simulink model "hvdcmay22"  (R2024b)
settings: Solver=VariableStepAuto  StartTime=0.0  StopTime=0.5  RelTol=1e-3
undefined symbols (not defined in the file): D1, Delta, lagging, pulse
libraries: spsThreePhaseTransformerTwoWindingsLib x4, spsUniversalBridgeLib x4, spsThreePhaseVIMeasurementLib x3, spsMeanLib x2, spsPLL3phLib x2, spsPulseGeneratorThyristor12PulseLib x2, spsSeriesRLCBranchLib x2, spsThreePhaseSourceLib x2, spsCurrentMeasurementLib x1, spsThreePhaseHarmonicFilterLib x1, spsVoltageMeasurementLib x1, sps_lib x1
settings Model: Creator=HP  LastModifiedBy=HP
settings DataIOCC: SignalLogging=off  ReturnWorkspaceOutputs=off

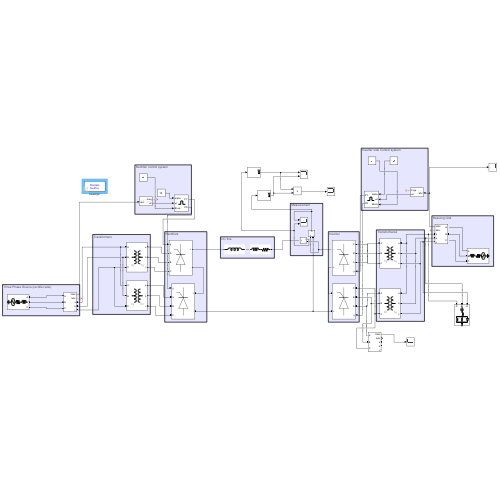
[thumbnail: Simulink's stored preview of the top-level diagram]
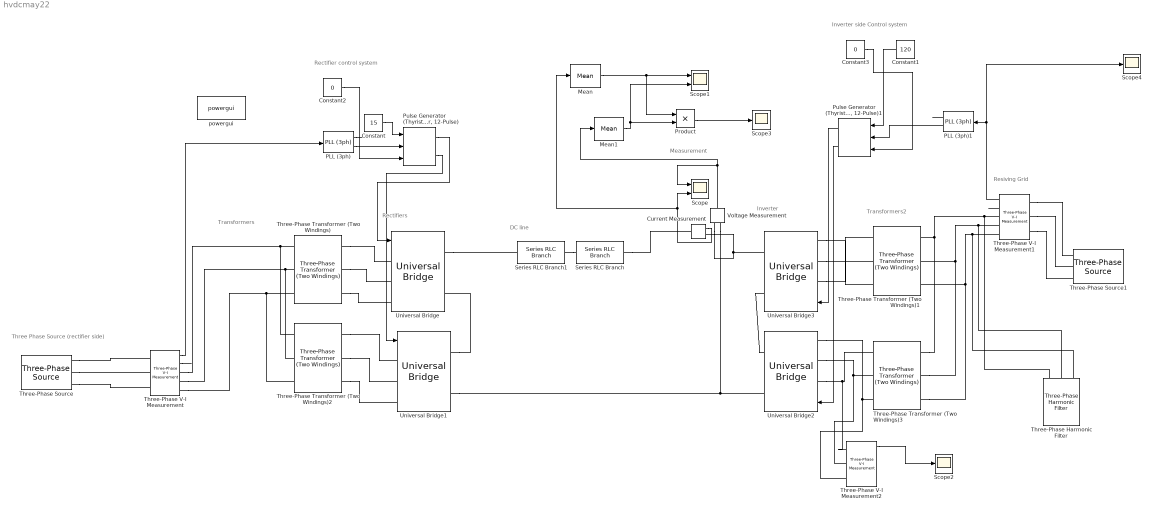
== system hvdcmay22 ==
  note: Transformers2
  note: Resiving Grid
  note: Inverter side Control system
  note: Measurement
  note: Inverter
  note: DC line
  note: Rectifiers
  note: Transformers
  note: Three Phase Source (rectifier side)
  note: Rectifier control system
  Constant : Constant  Value=15
  Constant1 : Constant  Value=120
  Constant2 : Constant  Value=0
  Constant3 : Constant  Value=0
  Current Measurement : spsCurrentMeasurementLib/Current Measurement  PhasorSimulation=off  OutputType=Complex  PSBequivalent=0
  Mean : spsMeanLib/Mean  Freq=60  Vinit=0  Ts=0
  Mean1 : spsMeanLib/Mean  Freq=60  Vinit=0  Ts=0
  PLL (3ph) : spsPLL3phLib/PLL (3ph)  Fmin=45  Par_Init=[0, 50]  ParK=[180, 3200, 1]  TcD=1e-4  MaxRateChangeFreq=12  FilterCutOffFreq=25  Ts=0  AGC=on
  PLL (3ph)1 : spsPLL3phLib/PLL (3ph)  Fmin=45  Par_Init=[0, 50]  ParK=[180, 3200, 1]  TcD=1e-4  MaxRateChangeFreq=12  FilterCutOffFreq=25  Ts=0  AGC=on
  Product : Product
  "Pulse Generator (Thyristor, 12-Pulse)" : spsPulseGeneratorThyristor12PulseLib/Pulse Generator (Thyristor, 12-Pulse)  GenType=12-pulse  Delta=D1 (lagging)  pwidth=60  Double_Pulse=off  Ts=0
      settings: LibrarySourceBlock=|
      | sps_lib/Power Electronics/Power Electronics Control/Pulse Generator
      | (Thyristor, 12-Pulse)
  "Pulse Generator (Thyristor, 12-Pulse)1" : spsPulseGeneratorThyristor12PulseLib/Pulse Generator (Thyristor, 12-Pulse)  GenType=12-pulse  Delta=D1 (lagging)  pwidth=60  Double_Pulse=off  Ts=0
  Scope : Scope  NumInputPorts=2
  Scope1 : Scope  NumInputPorts=2
  Scope2 : Scope
  Scope3 : Scope
  Scope4 : Scope
  Series RLC Branch : spsSeriesRLCBranchLib/Series RLC Branch  LConnTagsString=__new0  RConnTagsString=__new0  BranchType=RL  Resistance=10  Inductance=100e-3  SetiL0=off  InitialCurrent=0  Capacitance=1e-6  Setx0=off  InitialVoltage=0  Measurements=None
  Series RLC Branch1 : spsSeriesRLCBranchLib/Series RLC Branch  LConnTagsString=__new0  RConnTagsString=__new0  BranchType=L  Resistance=1  Inductance=0.5  SetiL0=off  InitialCurrent=0  Capacitance=1e-6  Setx0=off  InitialVoltage=0  Measurements=None
  Three-Phase Harmonic Filter : spsThreePhaseHarmonicFilterLib/Three-Phase Harmonic Filter  LConnTagsString=A|B|C  RConnTagsString=n  FilterType=Double-tuned  FilterConnection=Y (neutral)  ParNom=[230e3 50]  Qc=49e6  Fr=[5*60]  Frd=[11*60 13*60]  Q=16  Measurements=None
      settings: AttributesFormatString=\n
      settings: LibrarySourceBlock=|
      | sps_lib/Passives/Three-Phase
      | Harmonic Filter
  Three-Phase Transformer (Two Windings) : spsThreePhaseTransformerTwoWindingsLib/Three-Phase Transformer (Two Windings)  Winding1Connection=Yg  Winding2Connection=Yg  CoreType=Three single-phase transformers  SetSaturation=off  Hysteresis=off  DataFile='hysteresis'  SetInitialFlux=off  Measurements=None  UNITS=SI  NominalPower=[ 250e6 , 50 ]  Winding1=[230e3 4.3215 0.45854]  Winding2=[100e3 0.7938 0.084225]  Rm=1.0803e+06  Lm=2865.9  L0=2.8659  Saturation=[0 0;0.66655 1910.3;277.72 2419.6]  InitialFluxes=[1273.5 -1273.5 1114.3]  BreakLoop=off  DiscreteSolver=Trapezoidal iterative  DataType=on  TransfoNumber=1
  Three-Phase Transformer (Two Windings)1 : spsThreePhaseTransformerTwoWindingsLib/Three-Phase Transformer (Two Windings)  Winding1Connection=Yg  Winding2Connection=Yg  CoreType=Three single-phase transformers  SetSaturation=off  Hysteresis=off  DataFile='hysteresis'  SetInitialFlux=off  Measurements=None  UNITS=SI  NominalPower=[ 250e6 , 60 ]  Winding1=[100e3 0.000392 4.1592e-05]  Winding2=[230e3 0.7938 0.084225]  Rm=98  Lm=0.25995  L0=0.00025995  Saturation=[0 0;69.985 18.193;29161 23.044]  InitialFluxes=[12.129 -12.129 10.613]  BreakLoop=off  DiscreteSolver=Trapezoidal iterative  DataType=on  TransfoNumber=1
  Three-Phase Transformer (Two Windings)2 : spsThreePhaseTransformerTwoWindingsLib/Three-Phase Transformer (Two Windings)  Winding1Connection=Yg  Winding2Connection=Delta (D1)  CoreType=Three single-phase transformers  SetSaturation=off  Hysteresis=off  DataFile='hysteresis'  SetInitialFlux=off  Measurements=None  UNITS=SI  NominalPower=[ 250e6 , 60 ]  Winding1=[230e3 4.3218 0.45856]  Winding2=[100e3 2.3814 0.25267]  Rm=1.0804e+06  Lm=2866  L0=2.866  Saturation=[0 0;0.66653 1910.3;277.72 2419.7]  InitialFluxes=[1273.5 -1273.5 1114.3]  BreakLoop=off  DiscreteSolver=Trapezoidal iterative  DataType=on  TransfoNumber=1
  Three-Phase Transformer (Two Windings)3 : spsThreePhaseTransformerTwoWindingsLib/Three-Phase Transformer (Two Windings)  Winding1Connection=Delta (D1)  Winding2Connection=Yg  CoreType=Three single-phase transformers  SetSaturation=off  Hysteresis=off  DataFile='hysteresis'  SetInitialFlux=off  Measurements=None  UNITS=SI  NominalPower=[ 250e6 , 60 ]  Winding1=[100e3 4.3218 0.45856]  Winding2=[230e3 2.3814 0.25267]  Rm=1.0804e+06  Lm=2866  L0=2.866  Saturation=[0 0;0.66653 1910.3;277.72 2419.7]  InitialFluxes=[1273.5 -1273.5 1114.3]  BreakLoop=off  DiscreteSolver=Trapezoidal iterative  DataType=on  TransfoNumber=1
  Three-Phase V-I Measurement : spsThreePhaseVIMeasurementLib/Three-Phase V-I Measurement  VoltageMeasurement=phase-to-ground  SetLabelV=off  LabelV=Vabc  Vpu=off  VpuLL=off  CurrentMeasurement=yes  SetLabelI=off  LabelI=Iabc  Ipu=off  Pbase=100e6  Vbase=500e3  OutputType=Complex  PhasorSimulation=off  PSBequivalent=0
  Three-Phase V-I Measurement1 : spsThreePhaseVIMeasurementLib/Three-Phase V-I Measurement  VoltageMeasurement=phase-to-ground  SetLabelV=off  LabelV=Vabc  Vpu=off  VpuLL=off  CurrentMeasurement=yes  SetLabelI=off  LabelI=Iabc  Ipu=off  Pbase=100e6  Vbase=500e3  OutputType=Complex  PhasorSimulation=off  PSBequivalent=0
  Three-Phase V-I Measurement2 : spsThreePhaseVIMeasurementLib/Three-Phase V-I Measurement  VoltageMeasurement=phase-to-phase  SetLabelV=off  LabelV=Vabc  Vpu=off  VpuLL=off  CurrentMeasurement=yes  SetLabelI=off  LabelI=Iabc  Ipu=off  Pbase=100e6  Vbase=500e3  OutputType=Complex  PhasorSimulation=off  PSBequivalent=0
  Three-Phase Source : spsThreePhaseSourceLib/Three-Phase Source  InternalConnection=Yg  VoltagePhases=off  Voltage=230e3  PhaseAngle=0  Voltage_phases=[25e3 25e3 25e3]/sqrt(3)  PhaseAngles_phases=[0 -120 +120]  Frequency=50  NonIdealSource=on  SpecifyImpedance=off  Resistance=0.8929  Inductance=16.58e-3  ShortCircuitLevel=100e6  BaseVoltage=230e3  XRratio=7  BusType=swing  Pref=10e3  Qref=0  Prefabc=[10e3, 10e3, 10e3]  Qrefabc=[0, 0, 0]  Qmin=-inf  Qmax=inf
  Three-Phase Source1 : spsThreePhaseSourceLib/Three-Phase Source  InternalConnection=Yg  VoltagePhases=off  Voltage=200e3  PhaseAngle=0  Voltage_phases=[25e3 25e3 25e3]/sqrt(3)  PhaseAngles_phases=[0 -120 +120]  Frequency=50  NonIdealSource=on  SpecifyImpedance=off  Resistance=0.8929  Inductance=16.58e-3  ShortCircuitLevel=100e6  BaseVoltage=230e3  XRratio=7  BusType=swing  Pref=10e3  Qref=0  Prefabc=[10e3, 10e3, 10e3]  Qrefabc=[0, 0, 0]  Qmin=-inf  Qmax=inf
  Universal Bridge{,1..3} (4 alike) : spsUniversalBridgeLib/Universal Bridge  Arms=3  SnubberResistance=1e5  SnubberCapacitance=inf  Device=Thyristors  Ron=1e-3  Lon=0  ForwardVoltages="[  0  0  ]"  ForwardVoltage=0  GTOparameters=[ 10e-6 , 20e-6 ]  IGBTparameters=[ 1e-6 , 2e-6 ]  Measurements=None  Measurements_2=None  converterType=Rectifier
  Voltage Measurement : spsVoltageMeasurementLib/Voltage Measurement  PhasorSimulation=off  OutputType=Complex  PSBequivalent=0
  powergui : sps_lib/powergui  Priority=1  SimulationMode=Discrete  SampleTime=50e-6  frequency=60  Iterations=50  frequencyindice=50  Pbase=100e6  ErrMax=1e-4  UnitsV=kV  UnitsW=MW  buscounter=0  FunctionMessages=off  echomessages=off  EnableUseOfTLC=off  CurrentSourceSwitches=off  DisableSnubberDevices=off  DisableRonSwitches=off  DisableVfSwitches=off  DisplayEquations=off  AutomaticDiscreteSolvers=off  SolverType=Tustin/Backward Euler (TBE)  Interpol=off  ExternalGateDelay=off  methode=off  Ts=100  x0status=blocks  SPID=on  SwTol=0  HookPort=off  NonlinearTolerance=1e-4  nMaxIteration=100  ContinueOnMaxIteration=off  RestoreLinks=warning  ResistiveCurrentMeasurement=off  Frange=[0:2:500]  Ylog=off  Xlog=on  ShowGrid=off  save=off  variable=ZData  structure=0  ZoomFFT=off  StartTime=0.0  cycles=1  DisplayStyle=1  fundamental=60  FreqAxis=off  MaxFrequency=1000  frequencyindicesteady=1  RmsSteady=1  display=off
  wires:
  PLL (3ph)/1 -> ?
  Constant2/1 -> "Pulse Generator (Thyristor, 12-Pulse)"/3
  Constant/1 -> "Pulse Generator (Thyristor, 12-Pulse)"/1
  PLL (3ph)/2 -> "Pulse Generator (Thyristor, 12-Pulse)"/2
  Three-Phase V-I Measurement/1 -> PLL (3ph)/1
  Three-Phase V-I Measurement/2 -> ?
  "Pulse Generator (Thyristor, 12-Pulse)"/2 -> Universal Bridge1/1
  "Pulse Generator (Thyristor, 12-Pulse)"/1 -> Universal Bridge/1
  "Pulse Generator (Thyristor, 12-Pulse)1"/1 -> Universal Bridge3/1
  "Pulse Generator (Thyristor, 12-Pulse)1"/2 -> Universal Bridge2/1
  Voltage Measurement/1 -> Mean1/1, Scope/1
  Current Measurement/1 -> Mean/1, Scope/2
  PLL (3ph)1/2 -> "Pulse Generator (Thyristor, 12-Pulse)1"/2
  Three-Phase V-I Measurement1/1 -> Scope4/1, PLL (3ph)1/1
  PLL (3ph)1/1 -> ?
  Constant3/1 -> "Pulse Generator (Thyristor, 12-Pulse)1"/3
  Constant1/1 -> "Pulse Generator (Thyristor, 12-Pulse)1"/1
  Three-Phase V-I Measurement1/2 -> ?
  Mean/1 -> Product/1, Scope1/1
  Mean1/1 -> Scope1/2, Product/2
  Three-Phase V-I Measurement2/1 -> Scope2/1
  Product/1 -> Scope3/1
  connections:
  Three-Phase Source/RConn3 -- Three-Phase V-I Measurement/LConn3
  Three-Phase Source/RConn1 -- Three-Phase V-I Measurement/LConn1
  Three-Phase Source/RConn2 -- Three-Phase V-I Measurement/LConn2
  Three-Phase Transformer (Two Windings)2/LConn2 -- Three-Phase V-I Measurement/RConn2 -- Three-Phase Transformer (Two Windings)/LConn2
  Three-Phase Transformer (Two Windings)2/LConn1 -- Three-Phase Transformer (Two Windings)/LConn1 -- Three-Phase V-I Measurement/RConn1
  Three-Phase Transformer (Two Windings)2/LConn3 -- Three-Phase Transformer (Two Windings)/LConn3 -- Three-Phase V-I Measurement/RConn3
  Three-Phase Transformer (Two Windings)/RConn1 -- Universal Bridge/LConn1
  Three-Phase Transformer (Two Windings)/RConn2 -- Universal Bridge/LConn2
  Three-Phase Transformer (Two Windings)2/RConn1 -- Universal Bridge1/LConn1
  Three-Phase Transformer (Two Windings)/RConn3 -- Universal Bridge/LConn3
  Three-Phase Transformer (Two Windings)2/RConn2 -- Universal Bridge1/LConn2
  Three-Phase Transformer (Two Windings)2/RConn3 -- Universal Bridge1/LConn3
  Universal Bridge1/RConn1 -- Universal Bridge/RConn2
  Universal Bridge/RConn1 -- Series RLC Branch1/RConn1
  Series RLC Branch1/LConn1 -- Series RLC Branch/RConn1
  Universal Bridge3/RConn1 -- Universal Bridge2/RConn2
  Universal Bridge1/RConn2 -- Voltage Measurement/LConn2 -- Universal Bridge2/RConn1
  Current Measurement/RConn1 -- Voltage Measurement/LConn1 -- Universal Bridge3/RConn2
  Series RLC Branch/LConn1 -- Current Measurement/LConn1
  Three-Phase V-I Measurement1/LConn3 -- Three-Phase Source1/RConn3
  Three-Phase V-I Measurement1/LConn2 -- Three-Phase Source1/RConn2
  Three-Phase V-I Measurement1/LConn1 -- Three-Phase Source1/RConn1
  Universal Bridge2/LConn1 -- Three-Phase V-I Measurement2/LConn1 -- Three-Phase Transformer (Two Windings)3/LConn1
  Universal Bridge3/LConn2 -- Three-Phase Transformer (Two Windings)1/LConn2
  Universal Bridge3/LConn1 -- Three-Phase Transformer (Two Windings)1/LConn1
  Universal Bridge2/LConn3 -- Three-Phase V-I Measurement2/LConn3 -- Three-Phase Transformer (Two Windings)3/LConn3
  Universal Bridge3/LConn3 -- Three-Phase Transformer (Two Windings)1/LConn3
  Three-Phase Transformer (Two Windings)3/RConn2 -- Three-Phase Harmonic Filter/LConn2 -- Three-Phase V-I Measurement1/RConn2 -- Three-Phase Transformer (Two Windings)1/RConn2
  Universal Bridge2/LConn2 -- Three-Phase V-I Measurement2/LConn2 -- Three-Phase Transformer (Two Windings)3/LConn2
  Three-Phase Transformer (Two Windings)3/RConn1 -- Three-Phase Harmonic Filter/LConn1 -- Three-Phase V-I Measurement1/RConn1 -- Three-Phase Transformer (Two Windings)1/RConn1
  Three-Phase Transformer (Two Windings)1/RConn3 -- Three-Phase Harmonic Filter/LConn3 -- Three-Phase V-I Measurement1/RConn3 -- Three-Phase Transformer (Two Windings)3/RConn3
